simulink model "custom_pwm"  (R2017a)
settings: Solver=FixedStepDiscrete  StartTime=0.0  StopTime=inf  FixedStep=0.0002  RelTol=1e-3  EnableMultiTasking=on
libraries: slrtlib x1
settings Model: SimulationMode=external  Creator=Venkatraman  LastModifiedBy=awlloyd
settings SolverCC: EnableConcurrentExecution=on
settings DataIOCC: LimitDataPoints=on  SaveFormat=Array  LoggingToFile=on
settings OptimizationCC: BlockReduction=off  OptimizeBlockIOStorage=off  BufferReuse=off  GlobalBufferReuse=off  ExpressionFolding=off  LocalBlockOutputs=off  LifeSpan=inf
settings DebuggingCC: SolverPrmCheckMsg=warning  SFUnexpectedBacktrackingDiag=warning  SFNoUnconditionalDefaultTransitionDiag=warning  SFExecutionAtInitializationDiag=none
settings HardwareCC: ProdBitPerPointer=32  ProdBitPerSizeT=32  ProdBitPerPtrDiffT=32  ProdLargestAtomicFloat=None  ProdWordSize=32  ProdLongLongMode=on  ProdHWDeviceType=Generic->32-bit x86 compatible  TargetBitPerPointer=64  TargetBitPerSizeT=64  TargetBitPerPtrDiffT=64  TargetLongLongMode=on  TargetIntDivRoundTo=Zero  TargetEndianess=LittleEndian  TargetWordSize=64  TargetHWDeviceType=MATLAB Host
settings ModelReferenceCC: PropagateSignalLabelsOutOfModel=off
settings RTWCC: SystemTargetFile=slrt.tlc  TemplateMakefile=slrt_default_tmf  Description=Simulink Real-Time  RTWVerbose=off  RTWCompilerOptimization=on
settings SimulinkRealTimeCC: GeneratePreprocessorConditionals=Disable all
settings ConfigComp: CovMetricSettings=dw  CovHtmlReporting=on  CovSaveCumulativeToWorkspaceVar=on  CovSaveSingleToWorkspaceVar=on  CovExternalEMLEnable=off  CovSFcnEnable=off

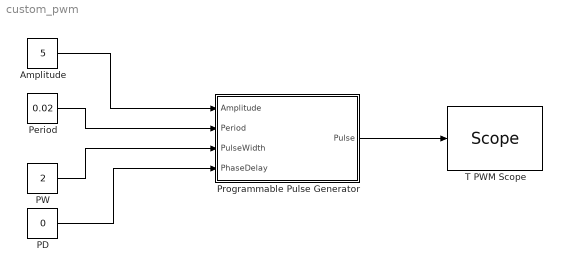
== system custom_pwm ==
  Amplitude : Constant  Value=5
  PD : Constant  Value=0
  PW : Constant  Value=2
  Period : Constant  Value=0.02
  Programmable Pulse Generator : Subsystem
  T PWM Scope : slrtlib/Displays and Logging/Scope   scopeno=1  scopetype=Target  autostart=on  viewmode=Graphical redraw  formatstr='%15.6f'  grid=on  ylimits=[0, 5]  nosamples=250  noprepostsamples=0  interleave=1  triggermode=FreeRun  triggersignal=1  trigsignalfromport=off  triggerlevel=0.0  triggerslope=Either  triggerscope=1  triggersample=0  filename=data.dat  mode=Lazy  writesize=512  autorestart=off  dynamicfilemode=off  maxwritefilesize=512*1024^2
  wires:
  Programmable Pulse Generator/1(Pulse) -> T PWM Scope/1
  PW/1 -> Programmable Pulse Generator/3(PulseWidth)
  PD/1 -> Programmable Pulse Generator/4(PhaseDelay)
  Period/1 -> Programmable Pulse Generator/2(Period)
  Amplitude/1 -> Programmable Pulse Generator/1(Amplitude)

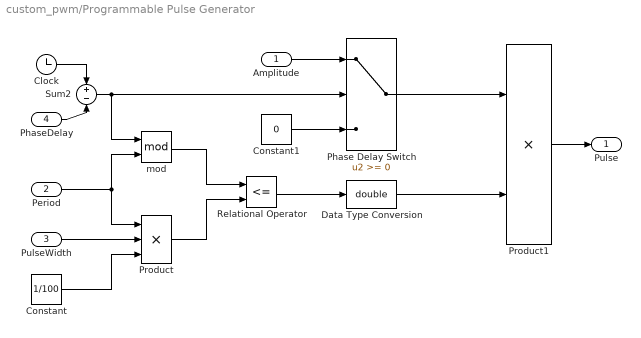
== system custom_pwm/Programmable Pulse Generator ==
  Amplitude : Inport
  Period : Inport  Port=2
  PulseWidth : Inport  Port=3
  PhaseDelay : Inport  Port=4
  Clock : Clock
  Constant : Constant  Value=1/100
  Constant1 : Constant  Value=0
  Data Type Conversion : DataTypeConversion  OutDataTypeStr=double
  Phase Delay Switch : Switch
  Product : Product  Inputs=3  RndMeth=Zero
  Product1 : Product  RndMeth=Zero
  Relational Operator : RelationalOperator  Operator=<=  RndMeth=Nearest
  Sum2 : Sum  Inputs=+-
  mod : Math  Operator=mod  SaturateOnIntegerOverflow=on
  Pulse : Outport
  wires:
  Phase Delay Switch/1 -> Product1/1
  Constant1/1 -> Phase Delay Switch/3
  Amplitude/1 -> Phase Delay Switch/1
  Sum2/1 -> Phase Delay Switch/2, mod/1
  PhaseDelay/1 -> Sum2/2
  Clock/1 -> Sum2/1
  Period/1 -> mod/2, Product/1
  mod/1 -> Relational Operator/1
  PulseWidth/1 -> Product/2
  Constant/1 -> Product/3
  Relational Operator/1 -> Data Type Conversion/1
  Data Type Conversion/1 -> Product1/2
  Product1/1 -> Pulse/1
  Product/1 -> Relational Operator/2
